simulink model "simulation"  (R2023b)
settings: Solver=VariableStepAuto  StartTime=0.0  StopTime=10.0  RelTol=1e-3
values from neighbouring files (symbols this model uses):
  cpp = 1000    [script.m]
  rop = 1.2    [script.m]
undefined symbols (not defined in the file or in its folder): Cv1, Cv2, k0, ks1, ks2
settings Model: Creator=igorkrzywda  LastModifiedBy=igorkrzywda

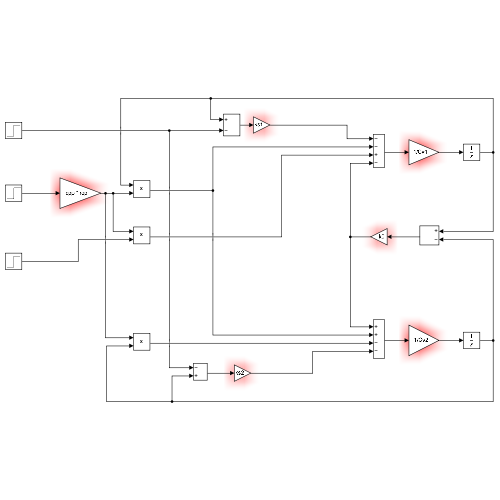
[thumbnail: Simulink's stored preview of the top-level diagram]
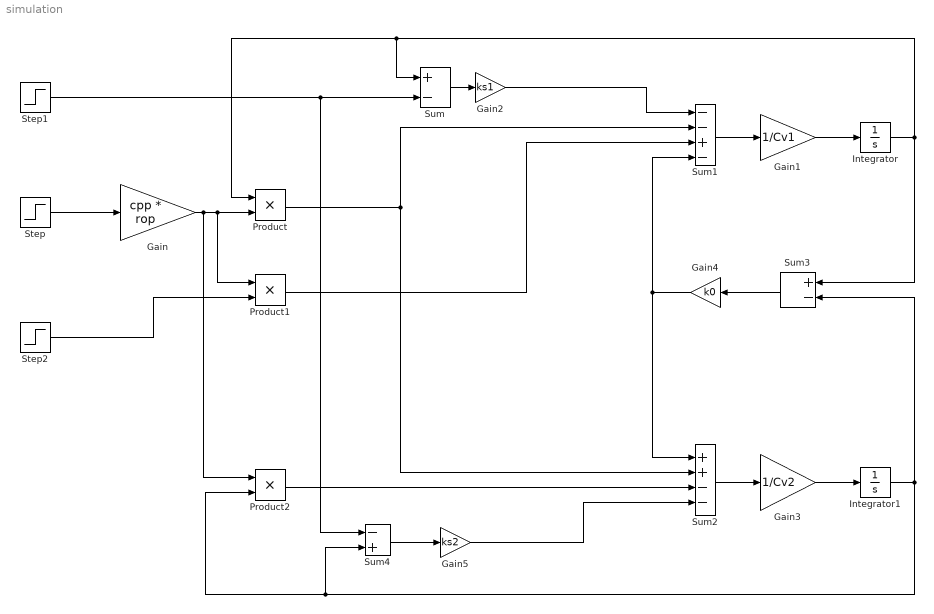
== system simulation ==
  Gain : Gain  Gain=cpp * rop
  Gain1 : Gain  Gain=1/Cv1
  Gain2 : Gain  Gain=ks1
  Gain3 : Gain  Gain=1/Cv2
  Gain4 : Gain  Gain=k0
  Gain5 : Gain  Gain=ks2
  Integrator : Integrator
  Integrator1 : Integrator
  Product : Product
  Product1 : Product
  Product2 : Product
  Step : Step  SampleTime=0
  Step1 : Step  SampleTime=0
  Step2 : Step  SampleTime=0
  Sum : Sum  Inputs=+-
  Sum1 : Sum  Inputs=--+-
  Sum2 : Sum  Inputs=++--
  Sum3 : Sum  Inputs=+-
  Sum4 : Sum  Inputs=-+
  wires:
  Step/1 -> Gain/1
  Sum1/1 -> Gain1/1
  Gain1/1 -> Integrator/1
  Integrator/1 -> Sum3/1, Sum/1, Product/1
  Step1/1 -> Sum4/1, Sum/2
  Sum/1 -> Gain2/1
  Gain2/1 -> Sum1/1
  Gain3/1 -> Integrator1/1
  Sum2/1 -> Gain3/1
  Integrator1/1 -> Sum3/2, Sum4/2, Product2/2
  Sum3/1 -> Gain4/1
  Gain4/1 -> Sum2/1, Sum1/4
  Gain/1 -> Product2/1, Product1/1, Product/2
  Product/1 -> Sum2/2, Sum1/2
  Product1/1 -> Sum1/3
  Step2/1 -> Product1/2
  Product2/1 -> Sum2/3
  Gain5/1 -> Sum2/4
  Sum4/1 -> Gain5/1
